simulink model "ASMC"  (R2021a)
settings: Solver=VariableStepAuto  StartTime=0.0  StopTime=inf  RelTol=1e-3
settings Model: Creator=Zicx  LastModifiedBy=Zicx
settings DataIOCC: SaveOutput=off  SaveTime=off

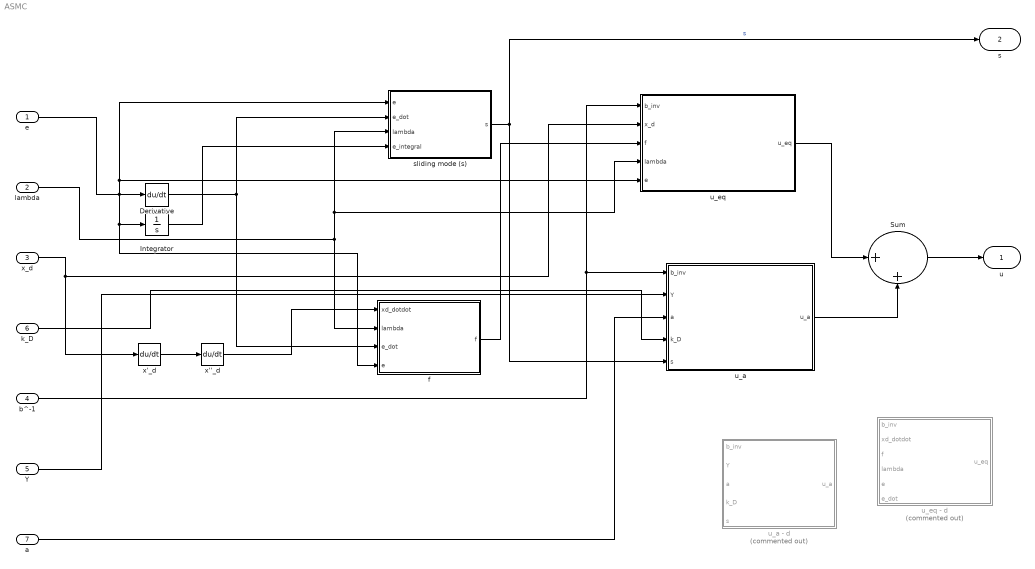
== system ASMC ==
  e : Inport  OutDataTypeStr=double  PortDimensions=[2 1]  SampleTime=0
  lambda : Inport  Port=2  OutDataTypeStr=double  PortDimensions=[2 2]
  x_d : Inport  Port=3  OutDataTypeStr=double  PortDimensions=2  SampleTime=0
  b^-1 : Inport  Port=4  OutDataTypeStr=double  PortDimensions=[2 2]  SampleTime=0
  Y : Inport  Port=5  OutDataTypeStr=double  PortDimensions=[2 4]  SampleTime=0
  k_D : Inport  Port=6  OutDataTypeStr=double  PortDimensions=[2 2]
  a : Inport  Port=7  OutDataTypeStr=double  PortDimensions=4  SampleTime=0
  Derivative : Derivative
  Integrator : Integrator
  Sum : Sum  Inputs=|++
  f : MATLAB Function  TreatAsAtomicUnit=on
  sliding mode (s) : MATLAB Function  TreatAsAtomicUnit=on
  u_a : Subsystem
  u_a - d : MATLAB Function  Commented=on  TreatAsAtomicUnit=on
  u_eq : Subsystem
  u_eq - d : MATLAB Function  Commented=on  TreatAsAtomicUnit=on
  x''_d : Derivative
  x'_d : Derivative
  u : Outport  OutDataTypeStr=double  PortDimensions=[2 1]  SampleTime=0
  s : Outport  Port=2  OutDataTypeStr=double  PortDimensions=2  SampleTime=0
  wires:
  e/1 -> Integrator/1, f/4(e), u_eq/5(e), sliding mode (s)/1(e), Derivative/1
  Derivative/1 -> f/3(e_dot), sliding mode (s)/2(e_dot)
  Integrator/1 -> sliding mode (s)/4(e_integral)
  lambda/1 -> f/2(lambda), sliding mode (s)/3(lambda), u_eq/4(lambda)
  x'_d/1 -> x''_d/1
  x_d/1 -> x'_d/1, u_eq/2(x_d)
  x''_d/1 -> f/1(xd_dotdot)
  Sum/1 -> u/1
  b^-1/1 -> u_a/1(b_inv), u_eq/1(b_inv)
  sliding mode (s)/1(s) -> s/1, u_a/5(s)  "s"
  f/1(f) -> u_eq/3(f)
  u_eq/1(u_eq) -> Sum/1
  u_a/1(u_a) -> Sum/2
  Y/1 -> u_a/2(Y)
  a/1 -> u_a/3(a)
  k_D/1 -> u_a/4(k_D)

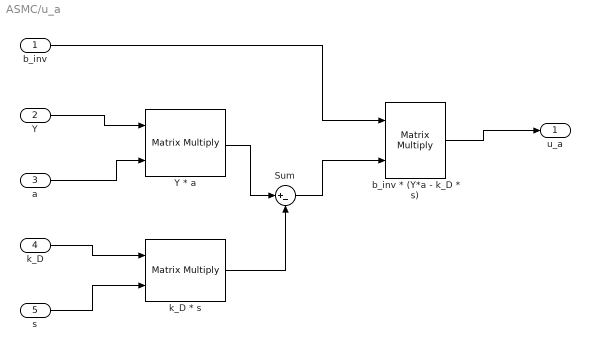
== system ASMC/u_a ==
  b_inv : Inport
  Y : Inport  Port=2  PortDimensions=[2 4]
  a : Inport  Port=3
  k_D : Inport  Port=4
  s : Inport  Port=5
  Sum : Sum  Inputs=|+-
  Y * a : Product  Multiplication=Matrix(*)
  b_inv * (Y*a - k_D * s) : Product  Multiplication=Matrix(*)
  k_D * s : Product  Multiplication=Matrix(*)
  u_a : Outport
  wires:
  b_inv * (Y*a - k_D * s)/1 -> u_a/1
  Sum/1 -> b_inv * (Y*a - k_D * s)/2
  b_inv/1 -> b_inv * (Y*a - k_D * s)/1
  k_D * s/1 -> Sum/2
  Y * a/1 -> Sum/1
  s/1 -> k_D * s/2
  k_D/1 -> k_D * s/1
  a/1 -> Y * a/2
  Y/1 -> Y * a/1

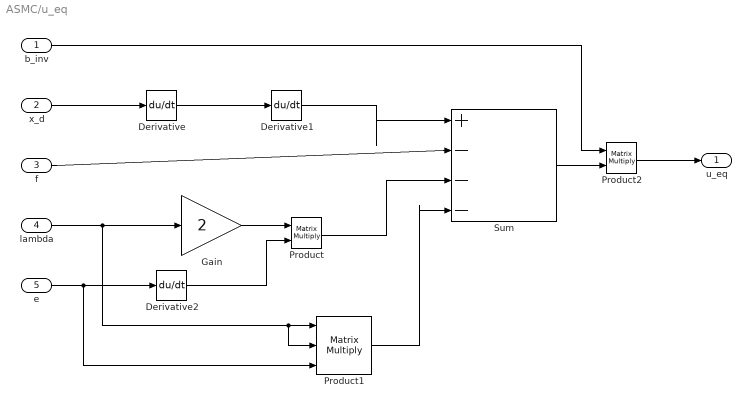
== system ASMC/u_eq ==
  b_inv : Inport
  x_d : Inport  Port=2
  f : Inport  Port=3  PortDimensions=[2 1]
  lambda : Inport  Port=4
  e : Inport  Port=5
  Derivative : Derivative
  Derivative1 : Derivative
  Derivative2 : Derivative
  Gain : Gain  Gain=2
  Product : Product  Multiplication=Matrix(*)
  Product1 : Product  Inputs=3  Multiplication=Matrix(*)
  Product2 : Product  Multiplication=Matrix(*)
  Sum : Sum  Inputs=|+---
  u_eq : Outport
  wires:
  Product2/1 -> u_eq/1
  Sum/1 -> Product2/2
  b_inv/1 -> Product2/1
  Product1/1 -> Sum/4
  Product/1 -> Sum/3
  Derivative2/1 -> Product/2
  Gain/1 -> Product/1
  lambda/1 -> Gain/1, Product1/1, Product1/2
  f/1 -> Sum/2
  Derivative1/1 -> Sum/1
  e/1 -> Derivative2/1, Product1/3
  x_d/1 -> Derivative/1
  Derivative/1 -> Derivative1/1

== matlab function ASMC/sliding mode (s) ==
  data: e input; s output; e_dot input; lambda input; e_integral input
function s = fcn(e, e_dot, lambda, e_integral)

s = e_dot + 2 * lambda * e + lambda * lambda * e_integral;

== matlab function ASMC/f ==
  data: xd_dotdot input; f output; lambda input; e_dot input; e input
function f = fcn(xd_dotdot, lambda, e_dot, e)

f = 5 * (xd_dotdot - 2 * lambda * e_dot - lambda^2 * e);

== matlab function ASMC/u_eq - d ==
  data: b_inv input; u_eq output; xd_dotdot input; f input; lambda input; e input; e_dot input
function u_eq = fcn(b_inv, xd_dotdot, f, lambda, e, e_dot)

% b_inv is 2x2
% xd_dotdot is 2x1
% f is 2x1
% lambda is 2x2
% e is 2x1
%e_dot is 2x1

u_eq = b_inv * (xd_dotdot - f - 2 * e_dot * lambda - lambda^2 * e);

== matlab function ASMC/u_a - d ==
  data: b_inv input; u_a output; Y input; a input; k_D input; s input
function u_a = fcn(b_inv, Y, a, k_D, s)

! b_inv is 2x2
! Y is 2x4
! a is 4x1
! k_D is k_D * I_2x2
! s is 2x1

u_a = b_inv * (Y * a - k_D * s);
